simulink model "Project_motor_speed_reader"  (R2023b)
settings: Solver=ode3  StartTime=0.0  StopTime=inf  FixedStep=0.001  RelTol=1e-3  EnableMultiTasking=on
libraries: arduinolib x3, eeGeneralControl x1, simulink_extras x1
settings Model: FPTRunName=Active  ExtModeTrigDuration=2  Creator=AHMED MOHSEN  LastModifiedBy=AHMED MOHSEN
settings SolverCC: AlgebraicLoopSolver=TrustRegion  AutoInsertRateTranBlk=on
settings DataIOCC: LimitDataPoints=on  SaveFormat=Array
settings OptimizationCC: ReuseModelBlockBuffer=off  ExpressionDepthLimit=2147483647  LifeSpan=Inf  MaxStackSize=64
settings DebuggingCC: UnderspecifiedInitializationDetection=Classic  MergeDetectMultiDrivingBlocksExec=none  FcnCallInpInsideContextMsg=warning  UnconnectedInputMsg=warning  UnconnectedOutputMsg=warning  UnconnectedLineMsg=warning  AllowSymbolicDim=off  StateNameClashWarn=warning  SFUnexpectedBacktrackingDiag=warning  SFNoUnconditionalDefaultTransitionDiag=warning  SFExecutionAtInitializationDiag=none  ArithmeticOperatorsInVariantConditions=warning
settings HardwareCC: ProdBitPerInt=16  ProdBitPerPointer=16  ProdBitPerSizeT=16  ProdBitPerPtrDiffT=16  ProdLargestAtomicFloat=None  ProdWordSize=8  ProdHWDeviceType=Atmel->AVR  UseEmbeddedCoderFeatures=off  UseSimulinkCoderFeatures=off
settings ModelReferenceCC: EnableRefExpFcnMdlSchedulingChecks=on  PropagateSignalLabelsOutOfModel=off
settings SFSimCC: SimUseLocalCustomCode=off  CustomCodeUndefinedFunction=UseInterfaceOnly
settings RTWCC: Description=Embedded Coder  SystemTargetFile=ert.tlc  HardwareBoard=Arduino Mega 2560  TemplateMakefile=ert_default_tmf  GenerateReport=on  RTWVerbose=off  RTWUseLocalCustomCode=off  Toolchain=Arduino AVR  BuildConfiguration=Faster Runs  LaunchReport=on
settings CodeAppCC: ForceParamTrailComments=on  OperatorAnnotations=on  StateflowObjectComments=on  MATLABSourceComments=on
settings ERTTargetCC: MultiwordLength=2048  ERTCustomFileBanners=off  SupportContinuousTime=on  SupportNonInlinedSFcns=on  RemoveResetFunc=off  ModelStepFunctionPrototypeControlCompliant=off
settings ConfigComp: CovMetricSettings=dw  CovSaveCumulativeToWorkspaceVar=on  CovSaveSingleToWorkspaceVar=on  CovExternalEMLEnable=off  CovSFcnEnable=off

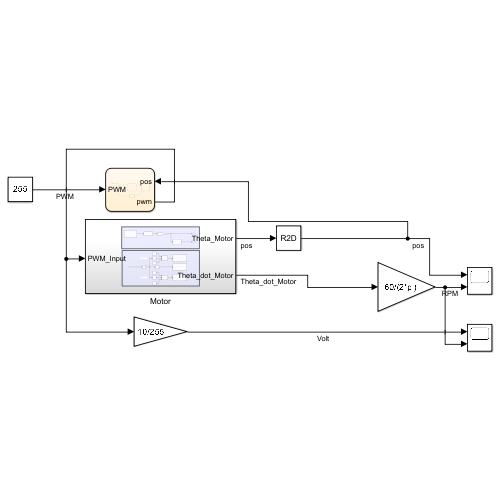
[thumbnail: Simulink's stored preview of the top-level diagram]
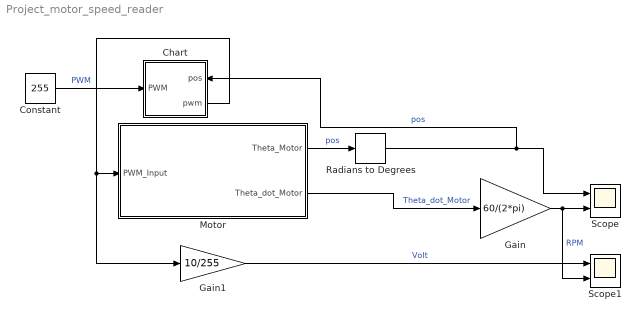
== system Project_motor_speed_reader ==
  Chart : Stateflow chart  TreatAsAtomicUnit=on
      settings: PortSchema="{\"entries\":[{\"content\":{\"sides\":[{\"content\":{\"connectorIds\":[\"In1\"]},\"type\":\"ConnectorPlacement.EquallySpacedRectSide\",\"uuid\":\"c5190a48-fc1c-4512-a04d-50b7311dfff4\"},{\"content\":{\"connectorIds\":[\"In2\",\"Out1\"],\"side\":\"RIGHT\"},\"type\":\"ConnectorPlacement.EquallySpacedRectSide\",\"uuid\":\"aa583b82-87b2-48c0-b5e7-9d4499e989ee\"},{\"content\":{\"side\":\"TOP\"},\"type\":\"ConnectorPlacement.EquallySpacedRectSide\",\"uuid\":\"8f13d879-6b07-4a86-a4b6-933503ee175d\"}]},\"type\":\"ConnectorPlacement.EquallySpacedConnector\",\"uuid\":\"eae082dc-271c-457e-b74b-f12769b84005\"}],\"packageUris\":[\"http://schema.mathworks.com/mf0/Connector/R2020b\"],\"version\":\"1.0\"}"
  Constant : Constant  Value=255
  Gain : Gain  Gain=60/(2*pi)
  Gain1 : Gain  Gain=10/255
  Motor : Subsystem
  Radians to Degrees : simulink_extras/Transformations/Radians to Degrees
  Scope : Scope  NumInputPorts=2
  Scope1 : Scope  NumInputPorts=2
  wires:
  Motor/2(Theta_dot_Motor) -> Gain/1  "Theta_dot_Motor"
  Motor/1(Theta_Motor) -> Radians to Degrees/1  "pos"
  Gain/1 -> Scope1/2, Scope/2  "RPM"
  Chart/1(pwm) -> Gain1/1, Motor/1(PWM_Input)
  Radians to Degrees/1 -> Chart/2(pos), Scope/1  "pos"
  Constant/1 -> Chart/1(PWM)  "PWM"
  Gain1/1 -> Scope1/1  "Volt"

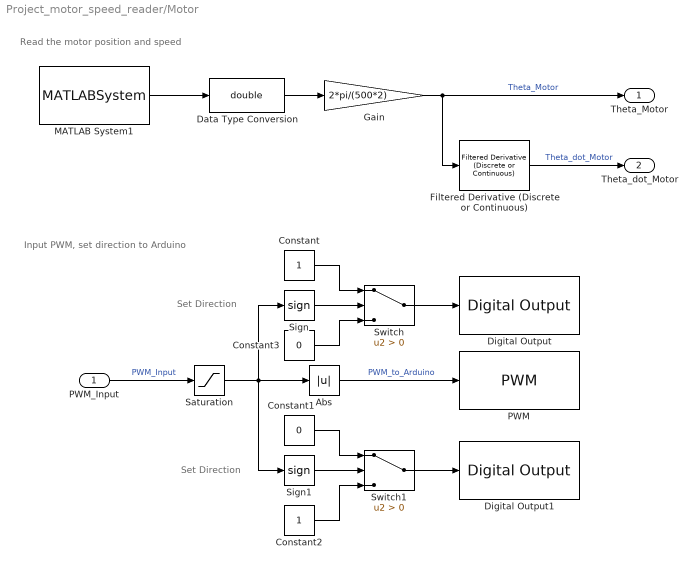
== system Project_motor_speed_reader/Motor ==
  note: Set Direction
  note: Input PWM, set direction to Arduino
  note: Read the motor position and speed
  note: Set Direction
  PWM_Input : Inport
  Abs : Abs  SaturateOnIntegerOverflow=off
  Constant : Constant
  Constant1 : Constant  Value=0
  Constant2 : Constant
  Constant3 : Constant  Value=0
  Data Type Conversion : DataTypeConversion  OutDataTypeStr=double  SaturateOnIntegerOverflow=off  RndMeth=Floor
  Digital Output : arduinolib/Digital Output  pinNumber=10  Direction=output  blockPlatform=arduino
  Digital Output1 : arduinolib/Digital Output  pinNumber=9  Direction=output  blockPlatform=arduino
  Filtered Derivative (Discrete or Continuous) : eeGeneralControl/Filtered Derivative (Discrete or Continuous)  K=1  T=0.001  B=inf  A=-inf  minRatio=10  init_option=Inherited from block input  x0=0  Ts=-1
      settings: LibrarySourceBlock=|
      | ee_sl_lib/General Control/Filtered Derivative
      | (Discrete or Continuous)
  Gain : Gain  Gain=2*pi/(500*2)
  MATLAB System1 : MATLABSystem  System=Encoder_arduino  Encoder=1  PinA=2  PinB=4  SampleTime=0.01
      mask Type: Encoder_arduino
      mask Display:
      | disp('Encoder');
      | port_label('output',1,'y');
  PWM : arduinolib/PWM  pinNumber=8  frequencyType=Default  desiredFrequency=490.2  achievableFrequency=490.2
  Saturation : Saturate  UpperLimit=255  LowerLimit=-255
  Sign : Signum
  Sign1 : Signum
  Switch : Switch  Criteria=u2 > Threshold  SaturateOnIntegerOverflow=off  InputSameDT=off
  Switch1 : Switch  Criteria=u2 > Threshold  SaturateOnIntegerOverflow=off  InputSameDT=off
  Theta_Motor : Outport
  Theta_dot_Motor : Outport  Port=2
  wires:
  MATLAB System1/1 -> Data Type Conversion/1
  Data Type Conversion/1 -> Gain/1
  Gain/1 -> Filtered Derivative (Discrete or Continuous)/1, Theta_Motor/1  "Theta_Motor"
  Filtered Derivative (Discrete or Continuous)/1 -> Theta_dot_Motor/1  "Theta_dot_Motor"
  PWM_Input/1 -> Saturation/1  "PWM_Input"
  Sign/1 -> Switch/2
  Constant/1 -> Switch/1
  Constant1/1 -> Switch1/1
  Sign1/1 -> Switch1/2
  Saturation/1 -> Abs/1, Sign1/1, Sign/1
  Constant2/1 -> Switch1/3
  Constant3/1 -> Switch/3
  Abs/1 -> PWM/1  "PWM_to_Arduino"
  Switch/1 -> Digital Output/1
  Switch1/1 -> Digital Output1/1

== stateflow chart Project_motor_speed_reader/Chart ==
  state cw
    entry:
    pwm=-PWM
  state ccw
    entry:
    pwm=PWM
  state cw1
    entry:
    pwm=-PWM/2
  state ccw1
    entry:
    pwm=PWM/2
  (default) -> cw
  cw -> ccw : [pos>=900 ]
  ccw -> cw1 : [pos<=0]
  ccw1 -> cw : [pos<=0]
  cw1 -> ccw1 : [pos>=900]
  data: PWM input; pos input; pwm output; t local =0
